simulink model "runfirst"  (Simulink 7.9)
settings: Solver=ode3  StartTime=0.0  StopTime=0.001  FixedStep=0.2  RelTol=0.02
values from neighbouring files (symbols this model uses):
  position_0 = [10; 15; -50]    [aerosonde_initialize.m]    (also in initial.m = [0; 5; 50])
  velocity_0 = [23; 0; 0]    [aerosonde_initialize.m]    (also in initial.m = [30; 0; 0])
undefined symbols (not defined in the file or in its folder): root_path
settings Model: Creator=Shihan Tissera  LastModifiedBy=Shihan Tissera

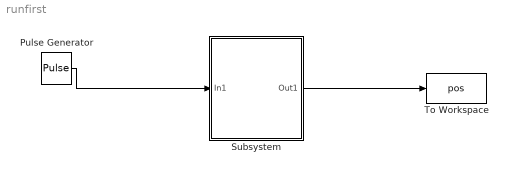
== system runfirst ==
  Pulse Generator : DiscretePulseGenerator  PulseType=Time based  Period=19  PulseWidth=20/19
  Subsystem : Subsystem
  To Workspace : ToWorkspace  VariableName=pos  SampleTime=-1
  wires:
  Pulse Generator/1 -> Subsystem/1(In1)
  Subsystem/1(Out1) -> To Workspace/1

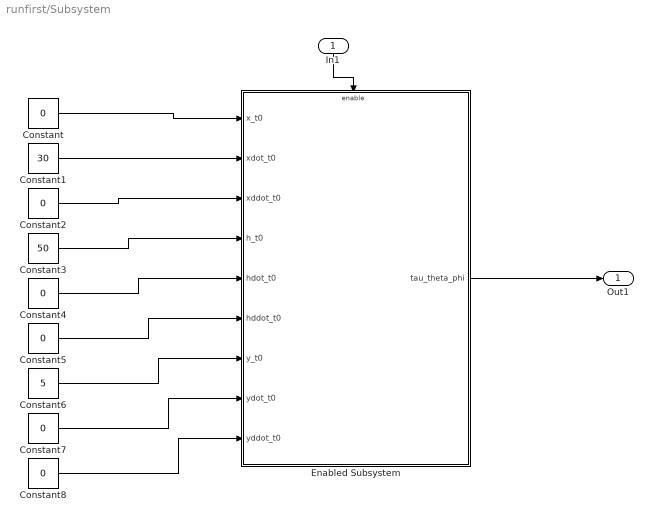
== system runfirst/Subsystem ==
  In1 : Inport
  Constant{,2,4..5,7..8} (6 alike) : Constant  Value=0
  Constant1 : Constant  Value=30
  Constant3 : Constant  Value=50
  Constant6 : Constant  Value=5
  Enabled Subsystem : Subsystem  TreatAsAtomicUnit=on
  Out1 : Outport
  wires:
  In1/1 -> Enabled Subsystem/Enable
  Enabled Subsystem/1(tau_theta_phi) -> Out1/1
  Constant/1 -> Enabled Subsystem/1(x_t0)
  Constant1/1 -> Enabled Subsystem/2(xdot_t0)
  Constant2/1 -> Enabled Subsystem/3(xddot_t0)
  Constant3/1 -> Enabled Subsystem/4(h_t0)
  Constant4/1 -> Enabled Subsystem/5(hdot_t0)
  Constant5/1 -> Enabled Subsystem/6(hddot_t0)
  Constant6/1 -> Enabled Subsystem/7(y_t0)
  Constant7/1 -> Enabled Subsystem/8(ydot_t0)
  Constant8/1 -> Enabled Subsystem/9(yddot_t0)

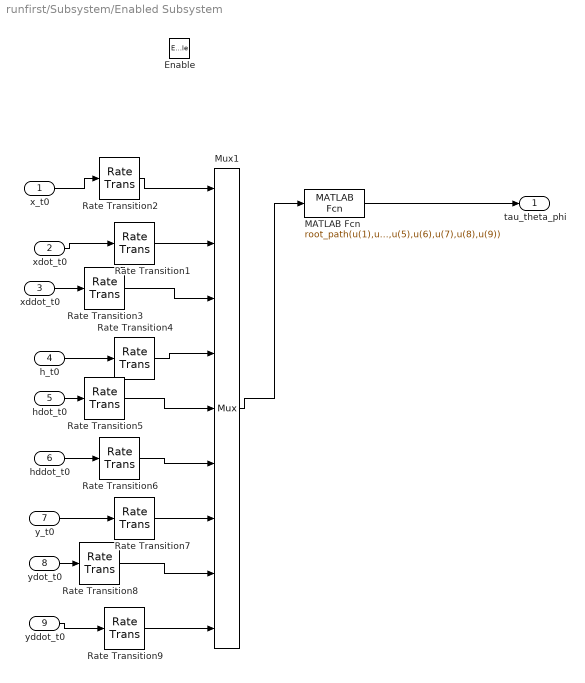
== system runfirst/Subsystem/Enabled Subsystem ==
  x_t0 : Inport
  xdot_t0 : Inport  Port=2
  xddot_t0 : Inport  Port=3
  h_t0 : Inport  Port=4
  hdot_t0 : Inport  Port=5
  hddot_t0 : Inport  Port=6
  y_t0 : Inport  Port=7
  ydot_t0 : Inport  Port=8
  yddot_t0 : Inport  Port=9
  Enable : EnablePort  StatesWhenEnabling=reset
  MATLAB Fcn : MATLABFcn  MATLABFcn=root_path(u(1),u(2),u(3),u(4),u(5),u(6),u(7),u(8),u(9))  OutputDimensions=[845 9]  Output1D=off
  Mux1 : Mux  Inputs=9
  Rate Transition1 : RateTransition  X0=velocity_0(1)
  Rate Transition2 : RateTransition  X0=position_0(1)
  Rate Transition3 : RateTransition
  Rate Transition4 : RateTransition  X0=position_0(3)
  Rate Transition5 : RateTransition  X0=velocity_0(3)
  Rate Transition6 : RateTransition
  Rate Transition7 : RateTransition  X0=position_0(2)
  Rate Transition8 : RateTransition  X0=velocity_0(2)
  Rate Transition9 : RateTransition
  tau_theta_phi : Outport
  wires:
  x_t0/1 -> Rate Transition2/1
  xdot_t0/1 -> Rate Transition1/1
  xddot_t0/1 -> Rate Transition3/1
  h_t0/1 -> Rate Transition4/1
  hdot_t0/1 -> Rate Transition5/1
  hddot_t0/1 -> Rate Transition6/1
  y_t0/1 -> Rate Transition7/1
  ydot_t0/1 -> Rate Transition8/1
  yddot_t0/1 -> Rate Transition9/1
  MATLAB Fcn/1 -> tau_theta_phi/1
  Mux1/1 -> MATLAB Fcn/1
  Rate Transition2/1 -> Mux1/1
  Rate Transition1/1 -> Mux1/2
  Rate Transition3/1 -> Mux1/3
  Rate Transition4/1 -> Mux1/4
  Rate Transition5/1 -> Mux1/5
  Rate Transition6/1 -> Mux1/6
  Rate Transition7/1 -> Mux1/7
  Rate Transition8/1 -> Mux1/8
  Rate Transition9/1 -> Mux1/9
